simulink model "rrmc21"  (R2020a)
settings: Solver=ode45  StartTime=0.0  StopTime=20.0  RelTol=1e-3  EnableMultiTasking=on
PreLoadFcn:
  | fprintf('*** Loading Puma560 model to workspace\n');
  | mdl_puma560
values from neighbouring files (symbols this model uses):
  planar3d = SerialLink(L)    [PUMA 260 Simulation.m]    (also in RoboticsSimAssign1CMC.m)
undefined symbols (not defined in the file or in its folder): DiscIntNeverNeededParam, qk, transl
libraries: roblocks x5, simulink x1
settings Model: ExtModeTrigMode=oneshot  ExtModeArmWhenConnect=off  Creator=pic  LastModifiedBy=mluser
settings DataIOCC: SaveFormat=Array  SignalLoggingSaveFormat=ModelDataLogs  ReturnWorkspaceOutputs=off
settings OptimizationCC: BlockReduction=off  BooleanDataType=off  ExpressionDepthLimit=2147483647  InitFltsAndDblsToZero=on  LifeSpan=inf
settings DebuggingCC: SaveWithParameterizedLinksMsg=none  UnderspecifiedInitializationDetection=Classic  MergeDetectMultiDrivingBlocksExec=none  SignalResolutionControl=TryResolveAllWithWarning  MultiTaskDSMMsg=warning  MultiTaskCondExecSysMsg=none  FcnCallInpInsideContextMsg=warning  StateNameClashWarn=warning  SFUnexpectedBacktrackingDiag=warning  SFNoUnconditionalDefaultTransitionDiag=warning  SFExecutionAtInitializationDiag=none  ArithmeticOperatorsInVariantConditions=warning
settings HardwareCC: ProdBitPerPointer=32  ProdBitPerSizeT=32  ProdBitPerPtrDiffT=32  ProdLargestAtomicFloat=None  ProdIntDivRoundTo=Undefined  ProdEndianess=Unspecified  ProdWordSize=32  ProdHWDeviceType=32-bit Generic  TargetUnknown=on
settings ModelReferenceCC: PropagateSignalLabelsOutOfModel=off
settings SFSimCC: SimUseLocalCustomCode=off  CustomCodeUndefinedFunction=UseInterfaceOnly
settings RTWCC: RTWUseLocalCustomCode=off
settings CodeAppCC: StateflowObjectComments=on
settings GRTTargetCC: TargetLangStandard=C89/C90 (ANSI)  ModelReferenceCompliant=off  CompOptLevelCompliant=off  CombineOutputUpdateFcns=off  MatFileLogging=off  GRTInterface=on
settings ConfigComp: CovMetricSettings=dw  CovHtmlReporting=on  CovSaveCumulativeToWorkspaceVar=on  CovSaveSingleToWorkspaceVar=on  CovExternalEMLEnable=off

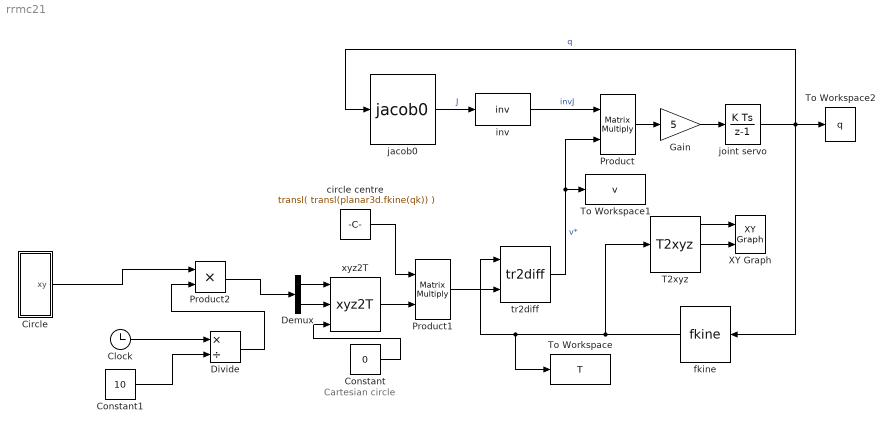
== system rrmc21 ==
  note: Cartesian circle
  Circle : Subsystem  mask{radius=5, freq=0.2}
      mask prompts: freq "Frequency (rev/s)"
  Clock : Clock
  Constant : Constant  Value=0
  Constant1 : Constant  Value=10
  Demux : Demux  Outputs=2
  Divide : Product  Inputs=*/
  Gain : Gain  Gain=5  SaturateOnIntegerOverflow=on  OutDataTypeStr=Inherit: Same as input  ParamDataTypeStr=Inherit: Same as input
  Product : Product  Multiplication=Matrix(*)  InputSameDT=on  RndMeth=Zero  SaturateOnIntegerOverflow=on  OutDataTypeStr=Inherit: Same as first input
  Product1 : Product  Multiplication=Matrix(*)  InputSameDT=on  RndMeth=Zero  SaturateOnIntegerOverflow=on  OutDataTypeStr=Inherit: Same as first input
  Product2 : Product
  T2xyz : roblocks/Transform Conversion/T2xyz
  To Workspace : ToWorkspace  VariableName=T  SampleTime=-1
  To Workspace1 : ToWorkspace  VariableName=v  SampleTime=-1
  To Workspace2 : ToWorkspace  VariableName=q  SampleTime=-1
  XY Graph : simulink/Sinks/XY Graph  xmin=-30  xmax=30  ymin=-30  ymax=30  st=-1
  circle centre : Constant  Value=transl( transl(planar3d.fkine(qk)) )
  fkine : roblocks/Kinematics/fkine  robot=planar3d
  inv : MATLABFcn  MATLABFcn=inv  Output1D=off
  "jacob0 " : roblocks/Kinematics/jacob0   robot=planar3d
  joint servo : DiscreteIntegrator  InitialCondition=qn'  SampleTime=0.05  ICPrevOutput=DiscIntNeverNeededParam  ICPrevScaledInput=DiscIntNeverNeededParam
  tr2diff : roblocks/Kinematics/tr2diff  robot=planar3d
  xyz2T : roblocks/Transform Conversion/xyz2T
  wires:
  joint servo/1 -> fkine/1, To Workspace2/1, "jacob0 "/1  "q"
  T2xyz/1 -> XY Graph/1
  T2xyz/2 -> XY Graph/2
  tr2diff/1 -> Product/2, To Workspace1/1  "v*"
  Demux/1 -> xyz2T/1
  "jacob0 "/1 -> inv/1  "J"
  Product/1 -> Gain/1
  inv/1 -> Product/1  "invJ"
  Gain/1 -> joint servo/1
  Demux/2 -> xyz2T/2
  Constant/1 -> xyz2T/3
  fkine/1 -> T2xyz/1, To Workspace/1, tr2diff/1
  xyz2T/1 -> Product1/2
  circle centre/1 -> Product1/1
  Product1/1 -> tr2diff/2
  Clock/1 -> Divide/1
  Constant1/1 -> Divide/2
  Circle/1(xy) -> Product2/1
  Divide/1 -> Product2/2
  Product2/1 -> Demux/1

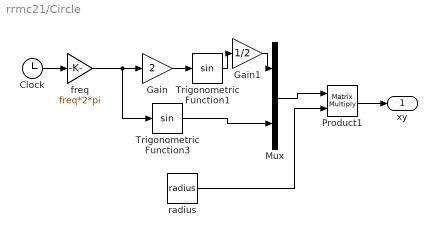
== system rrmc21/Circle ==
  Clock : Clock
  Gain : Gain  Gain=2
  Gain1 : Gain  Gain=1/2
  Mux : Mux  Inputs=2
  Product1 : Product  Multiplication=Matrix(*)  RndMeth=Zero
  Trigonometric Function1 : Trigonometry
  Trigonometric Function3 : Trigonometry
  freq : Gain  Gain=freq*2*pi
  radius : Constant  Value=radius
  xy : Outport
  wires:
  freq/1 -> Gain/1, Trigonometric Function3/1
  Product1/1 -> xy/1
  Clock/1 -> freq/1
  radius/1 -> Product1/2
  Mux/1 -> Product1/1
  Gain/1 -> Trigonometric Function1/1
  Trigonometric Function1/1 -> Gain1/1
  Gain1/1 -> Mux/1
  Trigonometric Function3/1 -> Mux/2
